simulink model "PLANTA_COMPLETA"  (R2024b)
settings: Solver=FixedStepAuto  StartTime=0.0  StopTime=inf  FixedStep=0.001  MaxStep=0.0005  RelTol=1e-4
undefined symbols (not defined in the file): A_hm, A_tm, at_breakpoints, at_max, b_ha, B_hm, b_ta, B_tm, bcx, bcy, bhd, bhEb, bhm, bt, btd, btm, btw, bwu, C_hm, C_tm, D_hm, D_tm, DiscIntNeverNeededParam, dl_h_ini, dx_l_ini, dx_t_ini, dx_td_ini, dxt_max, dy_l_ini, F01_a_t_max, F01_Ts1, F02_a_h_max, F02_Ts1, F03_a_h_max, F03_a_t_max, F03_dxt_max, F03_Ts1, Fhw_min, g, Hc, ih, it, Jhd_hEb, Jhm_hb, Jtd, Jtm_tb, K_hsa, K_hsia, K_tsa, K_tsia, Kcy, Kd_table, Ke_tita, Ke_w, kp_pos, Kp_table, kp_w, Ktw, kwu, l_breakpoints ... (+30)
libraries: simulink x13, spsEdgeDetectorLib x5, simulink_extras x2, dspsigops x2, vrlib x1, dspstat3 x1
(part 5 of 5)

== matlab function PLANTA_COMPLETA/Nivel 2 - Control Regulatorio + Obs/Controlador de balanceo/MATLAB Function ==
  data: xt0 input; Kp output; vt0 input; th0 input; w0 input; Ftw0 input; Mt0 input; ml0 input; l0 input; bt0 input; g0 input; Kd output
function [Kp, Kd] = jacob(xt0,vt0,th0,w0,Ftw0,Mt0,ml0,l0,bt0,g0)

syms xt vt th w Ftw real
syms Mt ml l bt g_sym real

%%Linealizacion Jacobiana 

% Estados y entrada
x = [xt; vt; th; w];
u = Ftw;

% Definiciones auxiliares
Dx  = Mt + ml*sin(th)^2;
Nx = Ftw - bt*vt + ml*l*w^2*sin(th) + ml*g_sym*sin(th)*cos(th);
Nth = -(Mt+ml*sin(th)^2)*g_sym*sin(th)-cos(th)*(Ftw-bt*vt+ml*l*w^2*sin(th)+ml*g_sym*sin(th)*cos(th));
Dth = l*(Mt+ml*sin(th)^2);

% Dinámica
f1 = vt;
f2 = Nx / Dx;
f3 = w;
f4 = Nth / Dth;

f = [f1; f2; f3; f4];

% Jacobianos
A = jacobian(f, x);
B = jacobian(f, u);

% (opcional) simplificación
A = simplify(A);
B = simplify(B);

% Modelo LPV evaluado en el punto de operacion
A0 = subs(A, {xt,vt,th,w,Ftw,Mt,ml,l,bt,g_sym}, {xt0,vt0,th0,w0,Ftw0,Mt0,ml0,l0,bt0,g0});
B0 = subs(B, {xt,vt,th,w,Ftw,Mt,ml,l,bt,g_sym}, {xt0,vt0,th0,w0,Ftw0,Mt0,ml0,l0,bt0,g0});

%% Buscamos la dinamica natural del sistema
% Autovalores de la matriz A0
lambda = eig(double(A0));

% Ordenar por real(lambda) (más cercano a 0 -> dominante)
[~, idx] = sort(real(lambda), 'descend'); % mayor real -> más lento (menos negativo)
lambda_ord = lambda(idx);

% Seleccionar el primer autovalor
lambda_dom = lambda_ord(1);

% Si es complejo (par), buscar su conjugado y calcular wn_la
if imag(lambda_dom) ~= 0
    sigma = real(lambda_dom);
    wd = abs(imag(lambda_dom));
    wn_la = sqrt(sigma^2 + wd^2);
    dseta = -sigma / wn_la;
else
    % polo real dominante
    sigma = real(lambda_dom);   % negativo para estable
    wn_la = abs(sigma);       % uso de |sigma| como medida de velocidad
    dseta = 1;              % no aplica exactamente, placeholder
end

%% Obtencion de Funcion de transferencia
syms Kp Kd s real

Gc = Kp+Kd*s;

% Selección de salida y vector que representa la acción de delta-theta
C = [0 1 0 0];            % salida y = delta v_t
a_theta = A0(:,3);        % influencia de delta theta como "entrada"

%Para encontrar la funcion de transferencia
SI_A0 = s*eye(4) - A0;
Gp = simplify( C * inv(SI_A0)* B(:,1));  % TF de la planta

% Separar numerador y denominador simbólicos (opcional)
% [numG, denG] = numden(Gp);
% numG = simplify(expand(numG));
% denG = simplify(expand(denG));

% 
% Gct = (1.7024e+04)/(s^2)+(2.2754e+04)/s+(1.0849e+04);
% Gct = simplify(Gct);
% 
% Gcb = Gp/(1+Gct*Gc*Gp); 

Gcb = Gp/(1+Gc*Gp)
Gcb = simplify(Gcb);
[~, denGcb] = numden(Gcb);
denGcb = expand(denGcb);

%% Diseño por amortiguamiento crítico
% Usamos una wn mayor a la de lazo abierto
wn = 1.5*wn_la;

% Polinomio dominante de segundo orden crítico
P_dom = s^2 + 2*wn*s + wn^2;

% Polos no dominantes (rápidos)
alpha = 5*wn;
beta = 6*wn;
P_des = expand(P_dom * (s + alpha) * (s + beta));

% Polinomio del lazo cerrado
P_lc = denGcb;

% % Igualación de coeficientes
% Pdiff = (expand(D_lc - D_des));
% coeffs_vec = coeffs(Pdiff, s);
% eqs = coeffs_vec == 0;

% Forma robusta: extraer polinomio en vector
% [~,D_des_p] = numden(D_des);
% poly_des = expand(D_des);

% Igualación por coeficientes (grado 4 -> 5 ecuaciones)
coeffs_lc = coeffs(P_lc,s,'All');
coeffs_des = coeffs(P_des, s, 'All');

% alinear longitudes rellenando con ceros si es necesario
nL = length(coeffs_lc); nD = length(coeffs_des);
n = max(nL, nD);
coeffs_lc = [zeros(1,n-nL), coeffs_lc];
coeffs_des = [zeros(1,n-nD), coeffs_des];

% formar sistema de ecuaciones (vectorial)
eqs = coeffs_lc - coeffs_des;
eqs = simplify(eqs);           % ecuaciones simbólicas

% Resolver simbólicamente Kp, Kd
sol = solve(eqs, [Kp Kd], 'Real', true);

% recoger soluciones posibles
Kp_sol = sol.Kp;
Kd_sol = sol.Kd;

% % Si solve devuelve múltiples soluciones, filtrar:
% found = false;
% Kp = NaN; Kd = NaN; wn = NaN;
%     for i = 1:length(wn_sym)
%         try
%             wn_i = double(wn_sym(i));
%             Kp_i = double(Kp_sym(i));
%             Kd_i = double(Kd_sym(i));
%         catch
%             continue;
%         end
%         if ~isreal(wn_i) || wn_i <= 0 || ~isreal(Kp_i) || ~isreal(Kd_i)
%             continue;
%         end
%         % comprobar estabilidad del lazo cerrado
%         poly_lc_sub = double(subs(poly_lc, {Kp,Kd,wn}, {Kp_i,Kd_i,wn_i}));
%         % opcional: comprobar raices todas en LHP
%         coeff_vec = sym2poly(poly_lc_sub);
%         if isempty(coeff_vec)
%             continue;
%         end
%         rts = roots(coeff_vec);
%         if all(real(rts) < 0)
%             Kp = Kp_i; Kd = Kd_i; wn = wn_i;
%             found = true;
%         end
%     end
% 
%     if ~found
%         warning('No se encontró solución válida para Kp,Kd,wn con los criterios dados.');
%     end

end

== matlab function PLANTA_COMPLETA/Nivel 2: Control Regulatorio1 ==
  data: Fhw input; T_tm output; T_hm output; dx_tref input; m_l input; BC input; dlh_ref input; l_h input; dl_h input; theta input; ddx_t_ref input; x_td input; dx_td input; xt_ref input; l_breakpoints parameter; ml_breakpoints parameter; at_breakpoints parameter; Kp_table parameter; Kd_table parameter
function [T_tm, T_hm]  = Nivel2(Fhw,dx_tref,m_l,BC,dlh_ref,l_h,dl_h,theta,ddx_t_ref, x_td, dx_td,xt_ref,l_breakpoints, ml_breakpoints, at_breakpoints, Kp_table, Kd_table)

%% PARAMETROS

% Datos generales
g = 9.80665;            % Aceleración gravitatoria [m/s^2]

% Accionamiento del Sistema de Izaje
tauhm = 1.0e-3;               % Constante de tiempo del modulador de torque en el motor [s]
Thm_Max = 20.0e3;             % Torque máximo de motorización/frenado regenerativo del motor [N*m]

% Accionamiento de Traslación del Carro
tautm = 1.0e-3;              % Constante de tiempo del modulador de torque (motor del carro) [s]
Ttm_Max = 4.0e3;             % Torque máximo de motorización/frenado regenerativo del motor [N*m]

% CN2 - DATOS GENERALES
T_s2=0.001; %Tiempo muestreo control nivel 2

% CN2 - PARAMETROS CONTROLADOR CARRO
b_ta = 1.084860000000000e+04;
K_tsa = 2.275381024560000e+04;
K_tsia = 1.702393005727008e+04;

% CN2 - PARAMETROS CONTROLADOR DE IZAJE
b_ha = -2.219636363636364e+04;
K_hsa = -8.441961938415557e+04;
K_hsia = -1.957032340849276e+05;

% CN2 - PARAMETROS OBSERVADOR CON CONTROL
%Observador
Ke_w = 10849.27;
Ke_tita = 209.27;
it = 30;
bt = 90;
Jtm_tb = 7;
Jtd = 1200;
rtd = 0.5;
Mt = 30000;
Ktw = 480000;
btw = 3000;
%Controlador
n = 2.5;
kp_pos = 0.15;
kp_w = n * kp_pos;


%% PROGRAM - MAIN

%VAR
persistent dx_td_obs_ant dxt_cp_ant ddxt_ant T_tm_out_ant;

if isempty(dx_td_obs_ant)
    dx_td_obs_ant = 0;
    dxt_cp_ant = 0;
    ddxt_ant = 0;
    T_tm_out_ant=0;
end

%BEGIN
if (BC==1)
    dx_tref_balanceo=controlBalanceo(m_l,l_h,ddxt_ant,ddx_t_ref,theta);
else
    dx_tref_balanceo=0;
end

[ddxt,dxt_pos,dx_td_obs]=observadorControl(T_tm_out_ant, x_td, xt_ref, theta, Fhw);

%Calculo de T_tm
T_tm_consig=controlCarro(dx_td,dx_tref+dx_tref_balanceo,b_ta,K_tsa,K_tsia);
T_tm_out=moduladorTorqueCarro(T_tm_consig);

%Calculo de T_hm
T_hm_consig=controlIzaje(dl_h,dlh_ref,b_ha,K_hsa,K_hsia);
T_hm_out=moduladorTorqueIzaje(T_hm_consig);

dxt_cp_ant = dxt_pos;
ddxt_ant = ddxt;
dx_td_obs_ant = dx_td_obs;
T_tm_out_ant = T_tm_out;
%OUTPUT
T_tm=T_tm_out;
T_hm=T_hm_out;

%% FUNCTION BLOCK - CONTROLADOR CARRO
function T_tm_consig=controlCarro(dx_t,dx_tref,b_ta,K_tsa,K_tsia)
    persistent error_prop_prev error_int_prev
    if isempty(error_prop_prev)
            error_prop_prev = 0;
            error_int_prev = 0;
    end
        error_t = dx_tref - dx_t;
        error_p = error_prop_prev + error_t*T_s2;
        error_i = error_int_prev + error_p*T_s2;
        T_tm_consig = K_tsia*error_i + K_tsa*error_p + b_ta*error_t;
        error_prop_prev = error_p;
        error_int_prev = error_i;
end
%% FUNCTION BLOCK - OBSERVADOR
function dx_td_obs=observador(x_td_real, T_tm_consigna)
    persistent int1_prev int2_prev 
    if isempty(int1_prev)
            int1_prev = 0;
            int2_prev = 0;
    end

   
    error_obs_pos = x_td_real - int2_prev;
    torque_in = T_tm_consigna*it*rtd/(Jtd+Jtm_tb*it^2);
    ddx_td_obs = Ke_w*error_obs_pos + torque_in;
    int1_prev = int1_prev + ddx_td_obs*T_s2;
    dx_td_obs = int1_prev ;
    int2_prev = int2_prev + (dx_td_obs + error_obs_pos*Ke_tita)* T_s2;
    
end
%% FUNCTION BLOCK - FUERZAS DE TENSION DE CABLE EN CARRO
function F_tw=fuerzaTension(dx_td_obs, x_td_real, x_t_obs, dx_t_obs)
    F_tw = (x_td_real-x_t_obs)*Ktw+(dx_td_obs-dx_t_obs)*btw;
end

%% FUNCTION BLOCK - FUERZAS DE TENSION DE CABLE EN CARRO
function [x_t_obs,dx_t_obs]=traslacCarro(F_tw, F_hw, theta)
    persistent int1_prev int2_prev 
    if isempty(int1_prev)
            int1_prev = 0;
            int2_prev = 0;
    end
    if isempty(F_tw)
            F_tw = 0;
    end
    
    dx_t_obs = int1_prev;
    x_t_obs = int2_prev;

    ddxt_obs = (F_tw+F_hw*sin(theta)*2-bt*dx_t_obs)*(1/Mt);

    int1_prev = int1_prev+ddxt_obs*T_s2;

    int2_prev = int2_prev+dx_t_obs*T_s2;

end

%% FUNCTION BLOCK - CONTROL DE POSICION
    function dx_t_pos=controlPosicion(x_t_obs, x_t_ref)
        persistent error_pos_ant der1_ant
        error_pos = x_t_ref-x_t_obs;
        if isempty(error_pos_ant)
            error_pos_ant = error_pos;
            der1_ant = 0;
        end

        if isempty(x_t_obs)
            x_t_obs=0;
        end

        sum1 = kp_pos*error_pos;
        sum2 = kp_w*(error_pos-error_pos_ant)/T_s2;
        dx_t_pos = sum1+sum2;

        error_pos_ant = error_pos;
    end
%% FUNCTION BLOCK - OBSERVADOR CON CONTROL
    function [ddx_t,dx_t_pos,dx_td_obs]=observadorControl(T_tm_consigna, x_td_real, x_t_ref, theta, F_hw)
        % Fuerza del cable
        persistent xt_ant dxt_ant 

        if isempty(xt_ant)
            xt_ant = 0;
            dxt_ant = 0;
        end

        xt=xt_ant;
        dxt=dxt_ant;
        
        dx_td_obs = observador(x_td_real, T_tm_consigna);
        F_tw = fuerzaTension(dx_td_obs, x_td_real, xt, dxt);
        
        [xt, dxt] = traslacCarro(F_tw, F_hw, theta);
        ddx_t = (dxt-dxt_ant)/T_s2;
        dx_t_pos=controlPosicion(xt, x_t_ref);
        
        xt_ant = xt;
        dxt_ant = dxt;

    end
%% FUNCTION BLOCK - CONTROLADOR BALANCEO
function dx_tref_balanceo=controlBalanceo(ml,lh,at,a_t_ref,theta)
    persistent error_p_prev theta_ant
    if isempty(error_p_prev)
    error_p_prev = 0;
    theta_ant = 0;
    end
    %Calculamos theta_ref
    theta_ref=atan(-a_t_ref/g);
    %Saturamos los input para evitar extrapolacion
    ml_sat = min(max(ml, ml_breakpoints(1)), ml_breakpoints(end));
    lh_sat = min(max(lh, l_breakpoints(1)), l_breakpoints(end));
    at_sat = min(max(at, at_breakpoints(1)), at_breakpoints(end));
    
    %Calculamos Kp y Kd
    Kp = interpn(ml_breakpoints,l_breakpoints, at_breakpoints, ...
                 Kp_table, ml_sat, lh_sat,at_sat, 'linear');
    
    Kd = interpn(ml_breakpoints,l_breakpoints, at_breakpoints, ...
                 Kd_table,ml_sat, lh_sat,  at_sat, 'linear');

    %Controlador
    error_p= theta_ref - theta;
    error_d=(theta-theta_ant)/T_s2;
    dx_tref_balanceo=Kp*0.3*error_p+Kd*(0.3)*error_d;

    error_p_prev = error_p;
    theta_ant = theta;
end
%% FUNCTION BLOCK - CONTROLADOR IZAJE
function T_hm_consig=controlIzaje(dl_h,dl_href,b_ha,K_hsa,K_hsia)
    persistent error_prop_prev error_int_prev
    if isempty(error_prop_prev)
            error_prop_prev = 0;
            error_int_prev = 0;
    end
        error_t = dl_href - dl_h;
        error_p = error_prop_prev + error_t*T_s2;
        error_i = error_int_prev + error_p*T_s2;
        T_hm_consig = K_hsia*error_i + K_hsa*error_p + b_ha*error_t;
        error_prop_prev = error_p;
        error_int_prev = error_i;
end
%% FUNCTION BLOCK - MODULADOR DE TORQUE EQUIVALENTE CARRO
function T_tm=moduladorTorqueCarro(T_tm_consig)
    persistent T_tm_ant
    
    if isempty(T_tm_ant)
    T_tm_ant = 0;
    end
    
    T_tm_lim = min(Ttm_Max, max(-Ttm_Max, T_tm_consig));
    
    alpha = exp(-T_s2/tautm);
    
    T_tm = alpha*T_tm_ant + (1 - alpha)*T_tm_lim;
    
    T_tm_ant = T_tm;
end
%% FUNCTION BLOCK - MODULADOR DE TORQUE EQUIVALENTE IZAJE
function T_hm=moduladorTorqueIzaje(T_hm_consig)
    persistent T_hm_ant
    
    if isempty(T_hm_ant)
    T_hm_ant = 0;
    end
    
    T_hm_lim = min(Thm_Max, max(-Thm_Max, T_hm_consig));
    
    alpha = exp(-T_s2/tauhm);
    
    T_hm = alpha*T_hm_ant + (1 - alpha)*T_hm_lim;
    
    T_hm_ant = T_hm;
end
end
